simulink model "QUESTION3"  (R2020a)
settings: Solver=VariableStepAuto  StartTime=0.0  StopTime=10.0  RelTol=1e-3
settings Model: Creator=anjal  LastModifiedBy=anjal

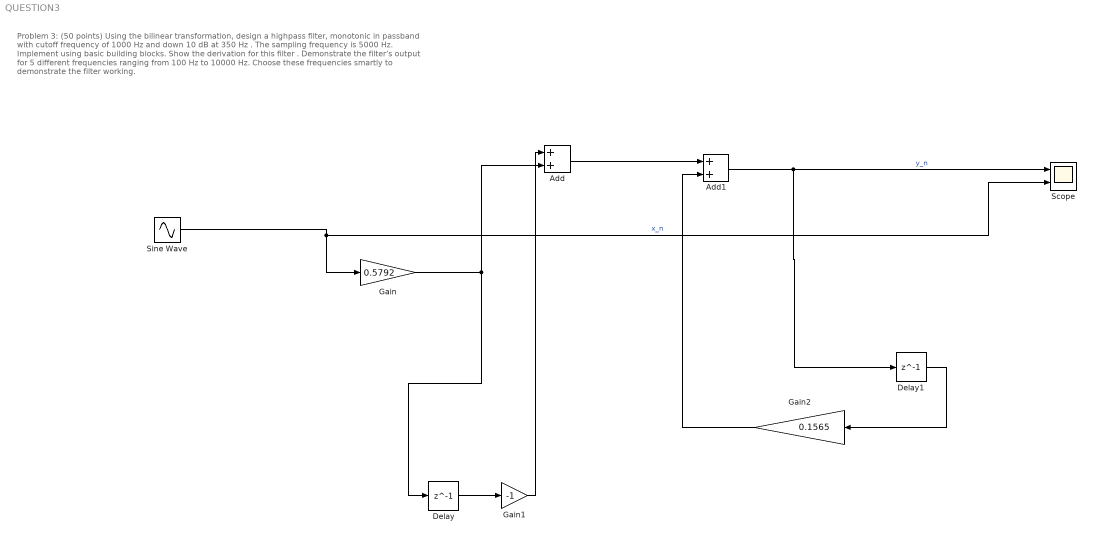
== system QUESTION3 ==
  note: Problem 3: (50 points) Using the bilinear transformation, design a highpass filter, monotonic in passband with cutoff frequency of 1000 Hz and down 10 dB at 350 Hz
      | . The sampling frequency is 5000 Hz. Implement using basic building blocks. Show the derivation for this filter
      | . Demonstrate the filter’s output for 5 different frequencies ranging from 100 Hz to 10000 Hz. Choose these frequencies smartly to demonstrate the filter working.
  Add : Sum
  Add1 : Sum
  Delay : Delay  DelayLength=1  InitialCondition=0
  Delay1 : Delay  DelayLength=1  InitialCondition=0
  Gain : Gain  Gain=0.5792
  Gain1 : Gain  Gain=-1
  Gain2 : Gain  Gain=0.1565
  Scope : Scope  NumInputPorts=2
  Sine Wave : Sin  SampleTime=0
  wires:
  Delay1/1 -> Gain2/1
  Add1/1 -> Delay1/1, Scope/1  "y_n"
  Delay/1 -> Gain1/1
  Add/1 -> Add1/1
  Gain/1 -> Delay/1, Add/2
  Sine Wave/1 -> Gain/1, Scope/2  "x_n"
  Gain1/1 -> Add/1
  Gain2/1 -> Add1/2
